simulink model "bolamagnetica_tp2"  (R2025a)
settings: Solver=VariableStepAuto  StartTime=0.0  StopTime=120  RelTol=1e-3
InitFcn:
  | m=0.5;
  | g=9.8;
  | R=2;
  | L=0.04;
  | K=8;
undefined symbols (not defined in the file or in its folder): dspblkCoreblockFVToolHelper, gcbh

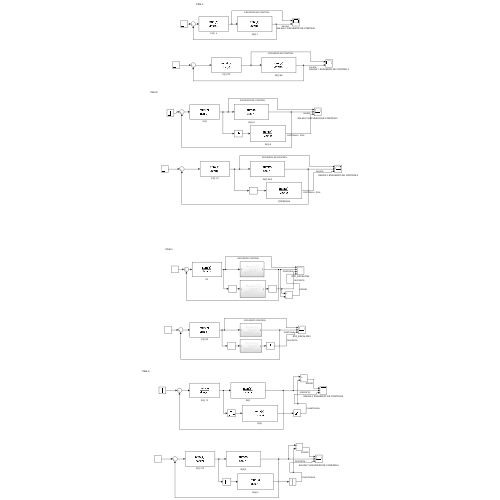
[thumbnail: Simulink's stored preview of the top-level diagram]
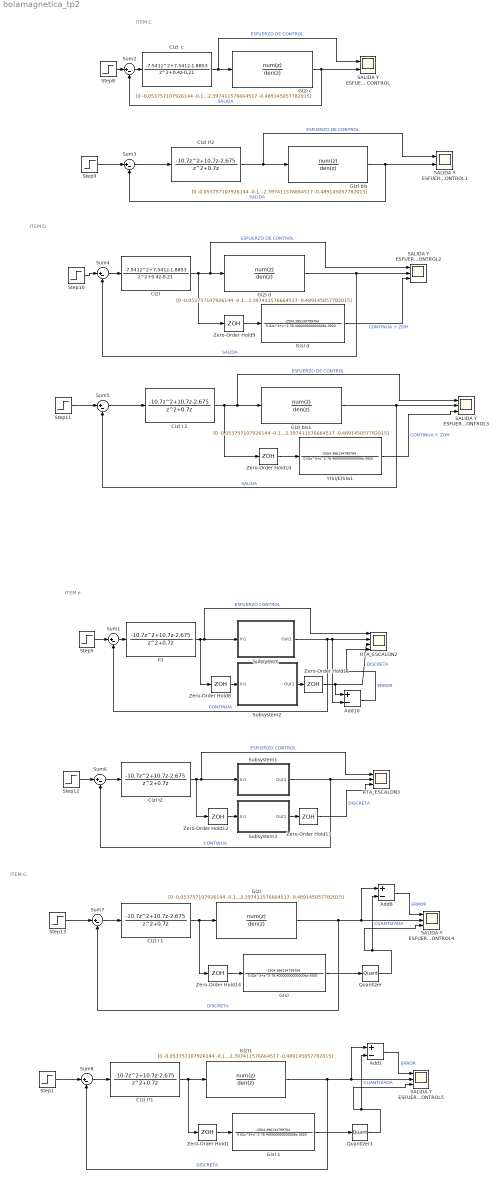
== system bolamagnetica_tp2 ==
  note: ITEM e
  note: ITEM G
  note: ITEM C
  note: ITEM D
  Add1 : Sum  Inputs=+-
  Add10 : Sum  Inputs=+-
  Add8 : Sum  Inputs=+-
  C(z) : DiscreteTransferFcn  LoadFcn=dspblkCoreblockFVToolHelper(gcbh,'load');  Numerator=[-7.541,7.541,-1.8853]  Denominator=[1,0.4,-0.21]  SampleTime=0.0143
      settings: CopyFcn=dspblkCoreblockFVToolHelper(gcbh,'copy');  DeleteFcn=dspblkCoreblockFVToolHelper(gcbh,'close');  ModelCloseFcn=dspblkCoreblockFVToolHelper(gcbh,'close');  PreSaveFcn=dspblkCoreblockFVToolHelper(gcbh,'presave');  PostSaveFcn=dspblkCoreblockFVToolHelper(gcbh,'postsave');  CloseFcn=dspblkCoreblockFVToolHelper(gcbh,'close');
  C(z)  c : DiscreteTransferFcn  LoadFcn=dspblkCoreblockFVToolHelper(gcbh,'load');  Numerator=[-7.541,7.541,-1.8853]  Denominator=[1,0.4,-0.21]  SampleTime=0.0143
      settings: CopyFcn=dspblkCoreblockFVToolHelper(gcbh,'copy');  DeleteFcn=dspblkCoreblockFVToolHelper(gcbh,'close');  ModelCloseFcn=dspblkCoreblockFVToolHelper(gcbh,'close');  PreSaveFcn=dspblkCoreblockFVToolHelper(gcbh,'presave');  PostSaveFcn=dspblkCoreblockFVToolHelper(gcbh,'postsave');  CloseFcn=dspblkCoreblockFVToolHelper(gcbh,'close');
  C(z) I 1 : DiscreteTransferFcn  LoadFcn=dspblkCoreblockFVToolHelper(gcbh,'load');  Numerator=[-10.7,10.7,-2.675]  Denominator=[1,0.7,0]  SampleTime=0.0143
      settings: CopyFcn=dspblkCoreblockFVToolHelper(gcbh,'copy');  DeleteFcn=dspblkCoreblockFVToolHelper(gcbh,'close');  ModelCloseFcn=dspblkCoreblockFVToolHelper(gcbh,'close');  PreSaveFcn=dspblkCoreblockFVToolHelper(gcbh,'presave');  PostSaveFcn=dspblkCoreblockFVToolHelper(gcbh,'postsave');  CloseFcn=dspblkCoreblockFVToolHelper(gcbh,'close');
  C(z) I 2 : DiscreteTransferFcn  LoadFcn=dspblkCoreblockFVToolHelper(gcbh,'load');  Numerator=[-10.7,10.7,-2.675]  Denominator=[1,0.7,0]  SampleTime=0.0143
      settings: CopyFcn=dspblkCoreblockFVToolHelper(gcbh,'copy');  DeleteFcn=dspblkCoreblockFVToolHelper(gcbh,'close');  ModelCloseFcn=dspblkCoreblockFVToolHelper(gcbh,'close');  PreSaveFcn=dspblkCoreblockFVToolHelper(gcbh,'presave');  PostSaveFcn=dspblkCoreblockFVToolHelper(gcbh,'postsave');  CloseFcn=dspblkCoreblockFVToolHelper(gcbh,'close');
  C(z) I2 : DiscreteTransferFcn  LoadFcn=dspblkCoreblockFVToolHelper(gcbh,'load');  Numerator=[-10.7,10.7,-2.675]  Denominator=[1,0.7,0]  SampleTime=0.0143
      settings: CopyFcn=dspblkCoreblockFVToolHelper(gcbh,'copy');  DeleteFcn=dspblkCoreblockFVToolHelper(gcbh,'close');  ModelCloseFcn=dspblkCoreblockFVToolHelper(gcbh,'close');  PreSaveFcn=dspblkCoreblockFVToolHelper(gcbh,'presave');  PostSaveFcn=dspblkCoreblockFVToolHelper(gcbh,'postsave');  CloseFcn=dspblkCoreblockFVToolHelper(gcbh,'close');
  C(z) I?1 : DiscreteTransferFcn  LoadFcn=dspblkCoreblockFVToolHelper(gcbh,'load');  Numerator=[-10.7,10.7,-2.675]  Denominator=[1,0.7,0]  SampleTime=0.0143
      settings: CopyFcn=dspblkCoreblockFVToolHelper(gcbh,'copy');  DeleteFcn=dspblkCoreblockFVToolHelper(gcbh,'close');  ModelCloseFcn=dspblkCoreblockFVToolHelper(gcbh,'close');  PreSaveFcn=dspblkCoreblockFVToolHelper(gcbh,'presave');  PostSaveFcn=dspblkCoreblockFVToolHelper(gcbh,'postsave');  CloseFcn=dspblkCoreblockFVToolHelper(gcbh,'close');
  C(z) I?2 : DiscreteTransferFcn  LoadFcn=dspblkCoreblockFVToolHelper(gcbh,'load');  Numerator=[-10.7,10.7,-2.675]  Denominator=[1,0.7,0]  SampleTime=0.0143
      settings: CopyFcn=dspblkCoreblockFVToolHelper(gcbh,'copy');  DeleteFcn=dspblkCoreblockFVToolHelper(gcbh,'close');  ModelCloseFcn=dspblkCoreblockFVToolHelper(gcbh,'close');  PreSaveFcn=dspblkCoreblockFVToolHelper(gcbh,'presave');  PostSaveFcn=dspblkCoreblockFVToolHelper(gcbh,'postsave');  CloseFcn=dspblkCoreblockFVToolHelper(gcbh,'close');
  "G(s) " : TransferFcn  Numerator=[-2504.396134799764]  Denominator=[0.02 1 -78.400000000000006 -3920]
  G(s) 1 : TransferFcn  Numerator=[-2504.396134799764]  Denominator=[0.02 1 -78.400000000000006 -3920]
  G(s) d : TransferFcn  Numerator=[-2504.396134799764]  Denominator=[0.02 1 -78.400000000000006 -3920]
  G(z) : DiscreteTransferFcn  LoadFcn=dspblkCoreblockFVToolHelper(gcbh,'load');  Numerator=[0 -0.053757107926144 -0.188445613408471 -0.037448542682446]  Denominator=[1 -3.345989984317626 2.397411576664517 -0.489145057782015]  SampleTime=0.0143
      settings: CopyFcn=dspblkCoreblockFVToolHelper(gcbh,'copy');  DeleteFcn=dspblkCoreblockFVToolHelper(gcbh,'close');  ModelCloseFcn=dspblkCoreblockFVToolHelper(gcbh,'close');  PreSaveFcn=dspblkCoreblockFVToolHelper(gcbh,'presave');  PostSaveFcn=dspblkCoreblockFVToolHelper(gcbh,'postsave');  CloseFcn=dspblkCoreblockFVToolHelper(gcbh,'close');
  G(z) bis : DiscreteTransferFcn  LoadFcn=dspblkCoreblockFVToolHelper(gcbh,'load');  Numerator=[0 -0.053757107926144 -0.188445613408471 -0.037448542682446]  Denominator=[1 -3.345989984317626 2.397411576664517 -0.489145057782015]  SampleTime=0.0143
      settings: CopyFcn=dspblkCoreblockFVToolHelper(gcbh,'copy');  DeleteFcn=dspblkCoreblockFVToolHelper(gcbh,'close');  ModelCloseFcn=dspblkCoreblockFVToolHelper(gcbh,'close');  PreSaveFcn=dspblkCoreblockFVToolHelper(gcbh,'presave');  PostSaveFcn=dspblkCoreblockFVToolHelper(gcbh,'postsave');  CloseFcn=dspblkCoreblockFVToolHelper(gcbh,'close');
  G(z) bis1 : DiscreteTransferFcn  LoadFcn=dspblkCoreblockFVToolHelper(gcbh,'load');  Numerator=[0 -0.053757107926144 -0.188445613408471 -0.037448542682446]  Denominator=[1 -3.345989984317626 2.397411576664517 -0.489145057782015]  SampleTime=0.0143
      settings: CopyFcn=dspblkCoreblockFVToolHelper(gcbh,'copy');  DeleteFcn=dspblkCoreblockFVToolHelper(gcbh,'close');  ModelCloseFcn=dspblkCoreblockFVToolHelper(gcbh,'close');  PreSaveFcn=dspblkCoreblockFVToolHelper(gcbh,'presave');  PostSaveFcn=dspblkCoreblockFVToolHelper(gcbh,'postsave');  CloseFcn=dspblkCoreblockFVToolHelper(gcbh,'close');
  G(z) c : DiscreteTransferFcn  LoadFcn=dspblkCoreblockFVToolHelper(gcbh,'load');  Numerator=[0 -0.053757107926144 -0.188445613408471 -0.037448542682446]  Denominator=[1 -3.345989984317626 2.397411576664517 -0.489145057782015]  SampleTime=0.0143
      settings: CopyFcn=dspblkCoreblockFVToolHelper(gcbh,'copy');  DeleteFcn=dspblkCoreblockFVToolHelper(gcbh,'close');  ModelCloseFcn=dspblkCoreblockFVToolHelper(gcbh,'close');  PreSaveFcn=dspblkCoreblockFVToolHelper(gcbh,'presave');  PostSaveFcn=dspblkCoreblockFVToolHelper(gcbh,'postsave');  CloseFcn=dspblkCoreblockFVToolHelper(gcbh,'close');
  G(z) d : DiscreteTransferFcn  LoadFcn=dspblkCoreblockFVToolHelper(gcbh,'load');  Numerator=[0 -0.053757107926144 -0.188445613408471 -0.037448542682446]  Denominator=[1 -3.345989984317626 2.397411576664517 -0.489145057782015]  SampleTime=0.0143
      settings: CopyFcn=dspblkCoreblockFVToolHelper(gcbh,'copy');  DeleteFcn=dspblkCoreblockFVToolHelper(gcbh,'close');  ModelCloseFcn=dspblkCoreblockFVToolHelper(gcbh,'close');  PreSaveFcn=dspblkCoreblockFVToolHelper(gcbh,'presave');  PostSaveFcn=dspblkCoreblockFVToolHelper(gcbh,'postsave');  CloseFcn=dspblkCoreblockFVToolHelper(gcbh,'close');
  G(z)1 : DiscreteTransferFcn  LoadFcn=dspblkCoreblockFVToolHelper(gcbh,'load');  Numerator=[0 -0.053757107926144 -0.188445613408471 -0.037448542682446]  Denominator=[1 -3.345989984317626 2.397411576664517 -0.489145057782015]  SampleTime=0.0143
      settings: CopyFcn=dspblkCoreblockFVToolHelper(gcbh,'copy');  DeleteFcn=dspblkCoreblockFVToolHelper(gcbh,'close');  ModelCloseFcn=dspblkCoreblockFVToolHelper(gcbh,'close');  PreSaveFcn=dspblkCoreblockFVToolHelper(gcbh,'presave');  PostSaveFcn=dspblkCoreblockFVToolHelper(gcbh,'postsave');  CloseFcn=dspblkCoreblockFVToolHelper(gcbh,'close');
  II1 : DiscreteTransferFcn  LoadFcn=dspblkCoreblockFVToolHelper(gcbh,'load');  Numerator=[-10.7,10.7,-2.675]  Denominator=[1,0.7,0]  SampleTime=0.0143
      settings: CopyFcn=dspblkCoreblockFVToolHelper(gcbh,'copy');  DeleteFcn=dspblkCoreblockFVToolHelper(gcbh,'close');  ModelCloseFcn=dspblkCoreblockFVToolHelper(gcbh,'close');  PreSaveFcn=dspblkCoreblockFVToolHelper(gcbh,'presave');  PostSaveFcn=dspblkCoreblockFVToolHelper(gcbh,'postsave');  CloseFcn=dspblkCoreblockFVToolHelper(gcbh,'close');
  Quantizer : Quantizer  QuantizationInterval=0.001123
  Quantizer1 : Quantizer  QuantizationInterval=0.001123
  RTA_ESCALON2 : Scope  NumInputPorts=4
      settings: ActiveDisplayYMinimum=-0.46260424416420359  ActiveDisplayYMaximum=4.1629368104432132  DataLoggingVariableName=ScopeData6
  RTA_ESCALON3 : Scope  NumInputPorts=3
      settings: ActiveDisplayYMinimum=-0.46254783812280875  ActiveDisplayYMaximum=4.16293054310528  DataLoggingVariableName=ScopeData10
  SALIDA Y ESFUERZO DE CONTROL : Scope  NumInputPorts=2
      settings: ActiveDisplayYMinimum=-0.14184096255304432  ActiveDisplayYMaximum=0.89951866297739913  DataLoggingVariableName=ScopeData5
  SALIDA Y ESFUERZO DE CONTROL1 : Scope  NumInputPorts=2
      settings: ActiveDisplayYMinimum=-0.24601206810588055  ActiveDisplayYMaximum=1.6791086129529251  DataLoggingVariableName=ScopeData7
  SALIDA Y ESFUERZO DE CONTROL{2..5} (4 alike) : Scope  NumInputPorts=3
      SALIDA Y ESFUERZO DE CONTROL2 settings: ActiveDisplayYMinimum=-0.14184096255304432  ActiveDisplayYMaximum=0.89951866297739913  DataLoggingVariableName=ScopeData8
      SALIDA Y ESFUERZO DE CONTROL3 settings: ActiveDisplayYMinimum=-0.24601485949452886  ActiveDisplayYMaximum=1.67913373545076  DataLoggingVariableName=ScopeData9
      SALIDA Y ESFUERZO DE CONTROL4 settings: ActiveDisplayYMinimum=-1.4130701561035646E+305  ActiveDisplayYMaximum=1.4130701561035646E+305  DataLoggingVariableName=ScopeData11
      SALIDA Y ESFUERZO DE CONTROL5 settings: ActiveDisplayYMinimum=-1.4130701561035646E+305  ActiveDisplayYMaximum=1.4130701561035646E+305
  Step{1,5,8..13} (8 alike) : Step  Time=0  After=0.005  SampleTime=0
  Subsystem : Subsystem
  Subsystem1 : Subsystem
  Subsystem2 : Subsystem
  Subsystem3 : Subsystem
  Sum{1..8} (8 alike) : Sum  Inputs=|+-
  Y(S)/E(S)a1 : TransferFcn  Numerator=[-2504.396134799764]  Denominator=[0.02 1 -78.400000000000006 -3920]
  Zero-Order Hold{1,8..14} (8 alike) : ZeroOrderHold  SampleTime=0.0143
  wires:
  II1/1 -> Zero-Order Hold8/1, RTA_ESCALON2/1, Subsystem/1(In1)  "ESFUERZO CONTROL"
  Step5/1 -> Sum1/1
  Sum1/1 -> II1/1
  Subsystem/1(Out1) -> Add10/2, RTA_ESCALON2/2, Sum1/2  "CONTINUA"
  Step8/1 -> Sum2/1
  Sum2/1 -> C(z)  c/1
  C(z)  c/1 -> G(z) c/1, SALIDA Y ESFUERZO DE CONTROL/1  "ESFUERZO DE CONTROL"
  G(z) c/1 -> SALIDA Y ESFUERZO DE CONTROL/2, Sum2/2  "SALIDA"
  G(z) bis/1 -> Sum3/2, SALIDA Y ESFUERZO DE CONTROL1/2  "SALIDA"
  C(z) I?2/1 -> G(z) bis/1, SALIDA Y ESFUERZO DE CONTROL1/1  "ESFUERZO DE CONTROL"
  Step9/1 -> Sum3/1
  Sum3/1 -> C(z) I?2/1
  Sum5/1 -> C(z) I 2/1
  C(z) I 2/1 -> Zero-Order Hold10/1, G(z) bis1/1, SALIDA Y ESFUERZO DE CONTROL3/1  "ESFUERZO DE CONTROL"
  G(z) bis1/1 -> Sum5/2, SALIDA Y ESFUERZO DE CONTROL3/2  "SALIDA"
  C(z)/1 -> G(z) d/1, SALIDA Y ESFUERZO DE CONTROL2/1, Zero-Order Hold9/1  "ESFUERZO DE CONTROL"
  Step11/1 -> Sum5/1
  G(z) d/1 -> SALIDA Y ESFUERZO DE CONTROL2/2, Sum4/2  "SALIDA"
  Step10/1 -> Sum4/1
  Sum4/1 -> C(z)/1
  C(z) I2/1 -> Zero-Order Hold12/1, RTA_ESCALON3/1, Subsystem1/1(In1)  "ESFUERZO CONTROL"
  Step12/1 -> Sum6/1
  Subsystem1/1(Out1) -> RTA_ESCALON3/2, Sum6/2  "CONTINUA"
  Sum6/1 -> C(z) I2/1
  Zero-Order Hold9/1 -> G(s) d/1
  G(s) d/1 -> SALIDA Y ESFUERZO DE CONTROL2/3  "CONTINUA + ZOH"
  Y(S)/E(S)a1/1 -> SALIDA Y ESFUERZO DE CONTROL3/3  "CONTINUA + ZOH"
  Zero-Order Hold10/1 -> Y(S)/E(S)a1/1
  Zero-Order Hold8/1 -> Subsystem2/1(In1)
  Zero-Order Hold11/1 -> Add10/1, RTA_ESCALON2/3  "DISCRETA"
  Subsystem2/1(Out1) -> Zero-Order Hold11/1
  Zero-Order Hold12/1 -> Subsystem3/1(In1)
  Subsystem3/1(Out1) -> Zero-Order Hold13/1
  Zero-Order Hold13/1 -> RTA_ESCALON3/3  "DISCRETA"
  G(z)/1 -> Sum7/2, Add8/1, SALIDA Y ESFUERZO DE CONTROL4/2  "DISCRETA"
  Step13/1 -> Sum7/1
  Sum7/1 -> C(z) I 1/1
  C(z) I 1/1 -> G(z)/1, Zero-Order Hold14/1
  Zero-Order Hold14/1 -> "G(s) "/1
  "G(s) "/1 -> Quantizer/1
  Quantizer/1 -> Add8/2, SALIDA Y ESFUERZO DE CONTROL4/3  "CUANTIZADA"
  Add8/1 -> SALIDA Y ESFUERZO DE CONTROL4/1  "ERROR"
  Add10/1 -> RTA_ESCALON2/4  "ERROR"
  Quantizer1/1 -> Add1/2, SALIDA Y ESFUERZO DE CONTROL5/3  "CUANTIZADA"
  Add1/1 -> SALIDA Y ESFUERZO DE CONTROL5/1  "ERROR"
  Step1/1 -> Sum8/1
  C(z) I?1/1 -> G(z)1/1, Zero-Order Hold1/1
  G(s) 1/1 -> Quantizer1/1
  Sum8/1 -> C(z) I?1/1
  G(z)1/1 -> Sum8/2, Add1/1, SALIDA Y ESFUERZO DE CONTROL5/2  "DISCRETA"
  Zero-Order Hold1/1 -> G(s) 1/1

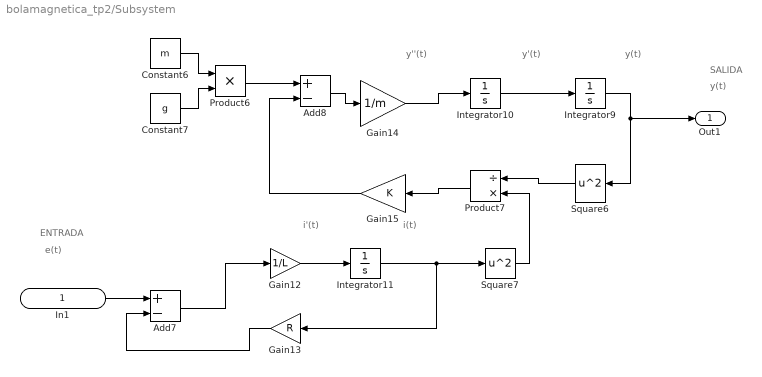
== system bolamagnetica_tp2/Subsystem ==
  note: SALIDA
  note: ENTRADA
  note: y(t)
  note: e(t)
  note: i'(t)
  note: i(t)
  note: y'(t)
  note: y(t)
  note: y''(t)
  In1 : Inport
  Add7 : Sum  Inputs=+-
  Add8 : Sum  Inputs=+-
  Constant6 : Constant  Value=m
  Constant7 : Constant  Value=g
  Gain12 : Gain  Gain=1/L
  Gain13 : Gain  Gain=R
  Gain14 : Gain  Gain=1/m
  Gain15 : Gain  Gain=K
  Integrator10 : Integrator
  Integrator11 : Integrator
  Integrator9 : Integrator  InitialCondition=0.005
  Product6 : Product
  Product7 : Product  Inputs=/*
  Square6 : Math  Operator=square  SignedPower=on
  Square7 : Math  Operator=square  SignedPower=on
  Out1 : Outport
  wires:
  Square6/1 -> Product7/1
  Gain14/1 -> Integrator10/1
  Integrator10/1 -> Integrator9/1
  Square7/1 -> Product7/2
  Constant7/1 -> Product6/2
  Product7/1 -> Gain15/1
  Constant6/1 -> Product6/1
  Integrator11/1 -> Gain13/1, Square7/1
  Product6/1 -> Add8/1
  Integrator9/1 -> Out1/1, Square6/1
  Gain15/1 -> Add8/2
  Gain12/1 -> Integrator11/1
  Add8/1 -> Gain14/1
  Gain13/1 -> Add7/2
  In1/1 -> Add7/1
  Add7/1 -> Gain12/1

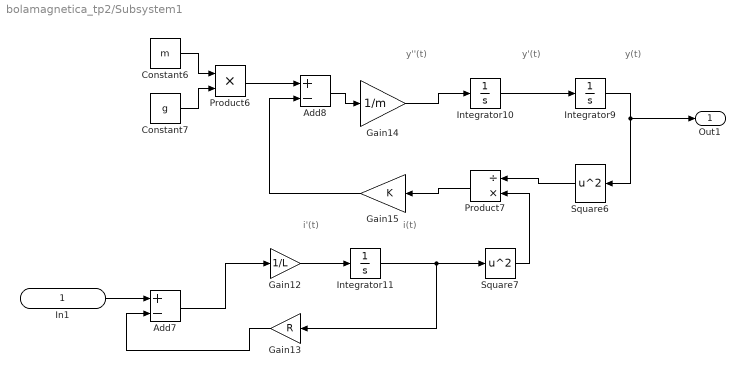
== system bolamagnetica_tp2/Subsystem1 ==
  note: i'(t)
  note: i(t)
  note: y'(t)
  note: y(t)
  note: y''(t)
  In1 : Inport
  Add7 : Sum  Inputs=+-
  Add8 : Sum  Inputs=+-
  Constant6 : Constant  Value=m
  Constant7 : Constant  Value=g
  Gain12 : Gain  Gain=1/L
  Gain13 : Gain  Gain=R
  Gain14 : Gain  Gain=1/m
  Gain15 : Gain  Gain=K
  Integrator10 : Integrator
  Integrator11 : Integrator
  Integrator9 : Integrator  InitialCondition=0.005
  Product6 : Product
  Product7 : Product  Inputs=/*
  Square6 : Math  Operator=square  SignedPower=on
  Square7 : Math  Operator=square  SignedPower=on
  Out1 : Outport
  wires:
  Square6/1 -> Product7/1
  Gain14/1 -> Integrator10/1
  Integrator10/1 -> Integrator9/1
  Square7/1 -> Product7/2
  Constant7/1 -> Product6/2
  Product7/1 -> Gain15/1
  Constant6/1 -> Product6/1
  Integrator11/1 -> Gain13/1, Square7/1
  Product6/1 -> Add8/1
  Integrator9/1 -> Out1/1, Square6/1
  Gain15/1 -> Add8/2
  Gain12/1 -> Integrator11/1
  Add8/1 -> Gain14/1
  Gain13/1 -> Add7/2
  In1/1 -> Add7/1
  Add7/1 -> Gain12/1

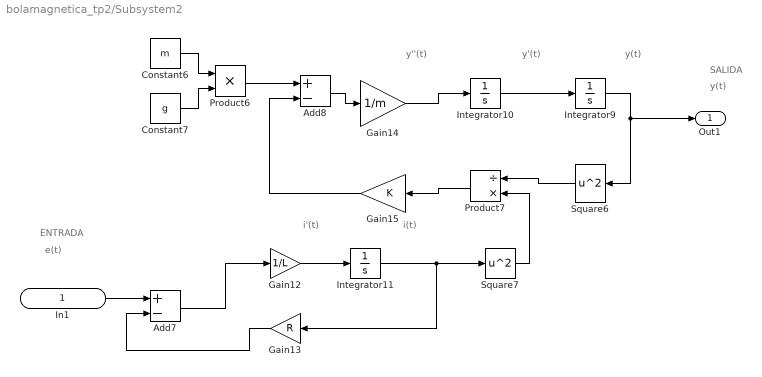
== system bolamagnetica_tp2/Subsystem2 ==
  note: SALIDA
  note: ENTRADA
  note: y(t)
  note: e(t)
  note: i'(t)
  note: i(t)
  note: y'(t)
  note: y(t)
  note: y''(t)
  In1 : Inport
  Add7 : Sum  Inputs=+-
  Add8 : Sum  Inputs=+-
  Constant6 : Constant  Value=m
  Constant7 : Constant  Value=g
  Gain12 : Gain  Gain=1/L
  Gain13 : Gain  Gain=R
  Gain14 : Gain  Gain=1/m
  Gain15 : Gain  Gain=K
  Integrator10 : Integrator
  Integrator11 : Integrator
  Integrator9 : Integrator  InitialCondition=0.005
  Product6 : Product
  Product7 : Product  Inputs=/*
  Square6 : Math  Operator=square  SignedPower=on
  Square7 : Math  Operator=square  SignedPower=on
  Out1 : Outport
  wires:
  Square6/1 -> Product7/1
  Gain14/1 -> Integrator10/1
  Integrator10/1 -> Integrator9/1
  Square7/1 -> Product7/2
  Constant7/1 -> Product6/2
  Product7/1 -> Gain15/1
  Constant6/1 -> Product6/1
  Integrator11/1 -> Gain13/1, Square7/1
  Product6/1 -> Add8/1
  Integrator9/1 -> Out1/1, Square6/1
  Gain15/1 -> Add8/2
  Gain12/1 -> Integrator11/1
  Add8/1 -> Gain14/1
  Gain13/1 -> Add7/2
  In1/1 -> Add7/1
  Add7/1 -> Gain12/1

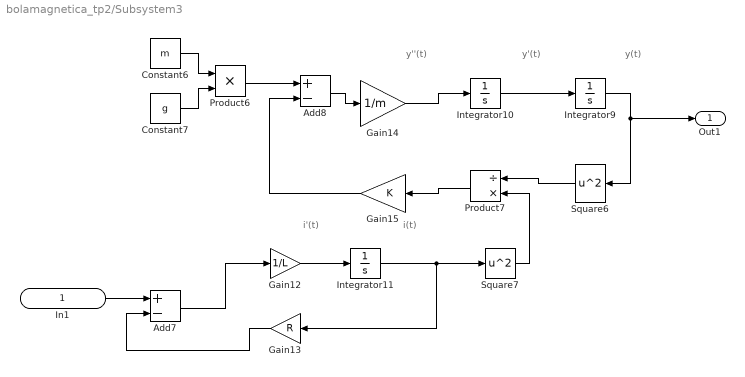
== system bolamagnetica_tp2/Subsystem3 ==
  note: i'(t)
  note: i(t)
  note: y'(t)
  note: y(t)
  note: y''(t)
  In1 : Inport
  Add7 : Sum  Inputs=+-
  Add8 : Sum  Inputs=+-
  Constant6 : Constant  Value=m
  Constant7 : Constant  Value=g
  Gain12 : Gain  Gain=1/L
  Gain13 : Gain  Gain=R
  Gain14 : Gain  Gain=1/m
  Gain15 : Gain  Gain=K
  Integrator10 : Integrator
  Integrator11 : Integrator
  Integrator9 : Integrator  InitialCondition=0.005
  Product6 : Product
  Product7 : Product  Inputs=/*
  Square6 : Math  Operator=square  SignedPower=on
  Square7 : Math  Operator=square  SignedPower=on
  Out1 : Outport
  wires:
  Square6/1 -> Product7/1
  Gain14/1 -> Integrator10/1
  Integrator10/1 -> Integrator9/1
  Square7/1 -> Product7/2
  Constant7/1 -> Product6/2
  Product7/1 -> Gain15/1
  Constant6/1 -> Product6/1
  Integrator11/1 -> Gain13/1, Square7/1
  Product6/1 -> Add8/1
  Integrator9/1 -> Out1/1, Square6/1
  Gain15/1 -> Add8/2
  Gain12/1 -> Integrator11/1
  Add8/1 -> Gain14/1
  Gain13/1 -> Add7/2
  In1/1 -> Add7/1
  Add7/1 -> Gain12/1
